simulink model "Stateflow_action"  (R2015b)
settings: Solver=VariableStepAuto  StartTime=0.0  StopTime=10.0  RelTol=1e-3
settings Model: Creator=amyyang  LastModifiedBy=amyyang

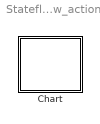
== system Stateflow_action ==
  Chart : Stateflow chart  TreatAsAtomicUnit=on

== stateflow chart Stateflow_action/Chart ==
  state A
  state B
  state A1
  state B1
  state Incorrect
  state B2
  state Incorrect1
  state B3
  A -> B : % 多个条件写在一行
      | [ condition1 && condition2 && condition3]
  B -> A : [ ( condition1 && condition2) || condition3]
  A1 -> B1 : % 分行时，操作符的位置都统一写在条件后面或者前面
      | [ condition1 &&...
      |   condition2 &&...
      |   condition3]
  B1 -> A1 : [ ( condition1 && condition2) ||...
      |     condition3]
  B2 -> Incorrect : % 使用了不同类型的运算符，没有使用括号把优先级显式表示出来
      | [  condition1 && condition2 ||...
      |     condition3]
  Incorrect1 -> B3 : % 超过四个运算符在同一行
      | [ condition1 && condition2 && condition3 && condition4]
